simulink model "sig_mod_block_6"  (R2019a)
settings: Solver=VariableStepAuto  StartTime=0.0  StopTime=10.0  RelTol=1e-3
undefined symbols (not defined in the file): mod_fcn, sig_in, sig_mod_enabled, sig_out
libraries: simulink x3
settings Model: Creator=a3bawa  LastModifiedBy=a3bawa

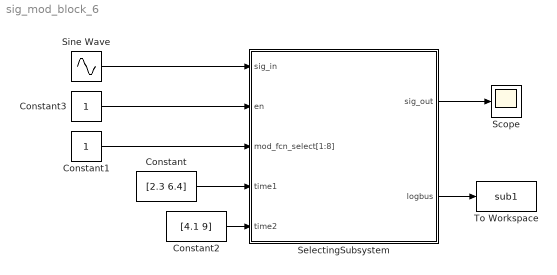
== system sig_mod_block_6 ==
  Constant : Constant  Value=[2.3 6.4]
  Constant1 : Constant
  Constant2 : Constant  Value=[4.1 9]
  Constant3 : Constant
  Scope : Scope
  SelectingSubsystem : Subsystem
  Sine Wave : Sin  SampleTime=0
  To Workspace : ToWorkspace  VariableName=sub1  SaveFormat=Timeseries  SampleTime=-1
  wires:
  Sine Wave/1 -> SelectingSubsystem/1(sig_in)
  Constant3/1 -> SelectingSubsystem/2(en)
  Constant1/1 -> SelectingSubsystem/3(mod_fcn_select[1:8])
  SelectingSubsystem/1(sig_out) -> Scope/1
  SelectingSubsystem/2(logbus) -> To Workspace/1
  Constant/1 -> SelectingSubsystem/4(time1)
  Constant2/1 -> SelectingSubsystem/5(time2)

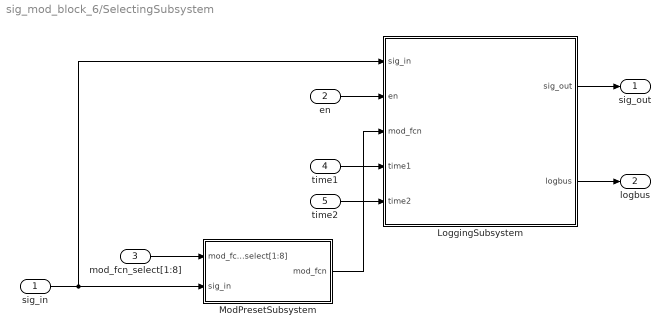
== system sig_mod_block_6/SelectingSubsystem ==
  sig_in : Inport
  en : Inport  Port=2
  mod_fcn_select[1:8] : Inport  Port=3
  time1 : Inport  Port=4
  time2 : Inport  Port=5
  LoggingSubsystem : Subsystem
  ModPresetSubsystem : Subsystem
  sig_out : Outport
  logbus : Outport  Port=2
  wires:
  sig_in/1 -> ModPresetSubsystem/2(sig_in), LoggingSubsystem/1(sig_in)
  en/1 -> LoggingSubsystem/2(en)
  LoggingSubsystem/1(sig_out) -> sig_out/1
  time1/1 -> LoggingSubsystem/4(time1)
  time2/1 -> LoggingSubsystem/5(time2)
  LoggingSubsystem/2(logbus) -> logbus/1
  mod_fcn_select[1:8]/1 -> ModPresetSubsystem/1(mod_fcn_select[1:8])
  ModPresetSubsystem/1(mod_fcn) -> LoggingSubsystem/3(mod_fcn)

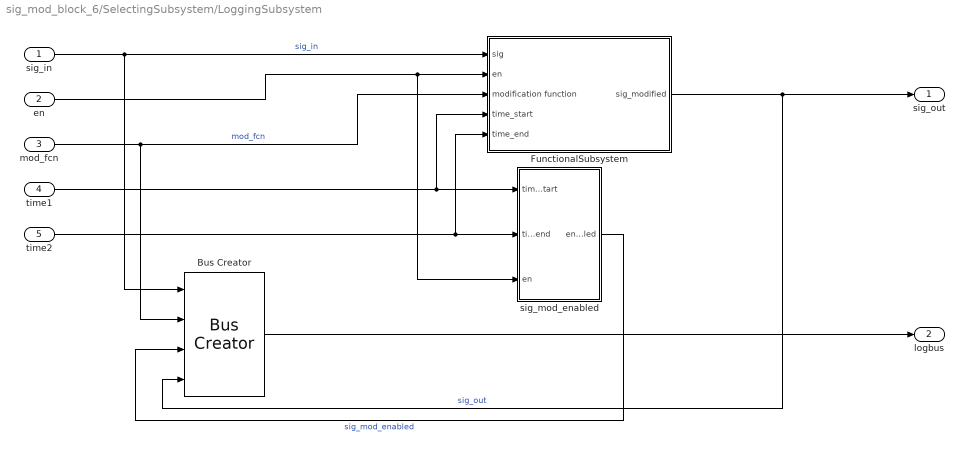
== system sig_mod_block_6/SelectingSubsystem/LoggingSubsystem ==
  sig_in : Inport
  en : Inport  Port=2
  mod_fcn : Inport  Port=3
  time1 : Inport  Port=4
  time2 : Inport  Port=5
  Bus Creator : BusCreator  Inputs=sig_in,mod_fcn,sig_mod_enabled,sig_out
  FunctionalSubsystem : Subsystem  TreatAsAtomicUnit=on
  sig_mod_enabled : Subsystem
  sig_out : Outport
  logbus : Outport  Port=2
  wires:
  FunctionalSubsystem/1(sig_modified) -> sig_out/1, Bus Creator/4  "sig_out"
  sig_in/1 -> FunctionalSubsystem/1(sig), Bus Creator/1  "sig_in"
  en/1 -> FunctionalSubsystem/2(en), sig_mod_enabled/3(en)
  sig_mod_enabled/1(enabled) -> Bus Creator/3  "sig_mod_enabled"
  mod_fcn/1 -> FunctionalSubsystem/3(modification function), Bus Creator/2  "mod_fcn"
  time1/1 -> sig_mod_enabled/1(time_start), FunctionalSubsystem/4(time_start)
  time2/1 -> FunctionalSubsystem/5(time_end), sig_mod_enabled/2(time_end)
  Bus Creator/1 -> logbus/1

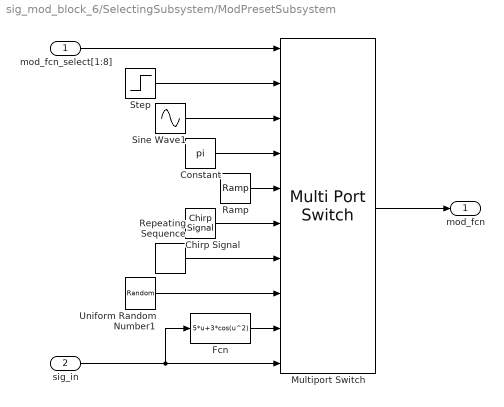
== system sig_mod_block_6/SelectingSubsystem/ModPresetSubsystem ==
  mod_fcn_select[1:8] : Inport
  sig_in : Inport  Port=2
  Chirp Signal : simulink/Sources/Chirp Signal  f1=1  T=10  f2=1000
  Constant : Constant  Value=pi
  Fcn : Fcn  Expr=5*u+3*cos(u^2)
  Multiport Switch : MultiPortSwitch  Inputs=8  DataPortForDefault=Additional data port  DiagnosticForDefault=Warning
  Ramp : simulink/Sources/Ramp  slope=1  start=5  InitialOutput=0
  Repeating Sequence : simulink/Sources/Repeating Sequence  rep_seq_t=[0 2]  rep_seq_y=[0 1]
  Sine Wave1 : Sin  Frequency=1000  SampleTime=0
  Step : Step  Time=5  SampleTime=0
  Uniform Random Number1 : UniformRandomNumber  SampleTime=0.1
  mod_fcn : Outport
  wires:
  mod_fcn_select[1:8]/1 -> Multiport Switch/1
  Step/1 -> Multiport Switch/2
  Chirp Signal/1 -> Multiport Switch/6
  sig_in/1 -> Fcn/1, Multiport Switch/10
  Fcn/1 -> Multiport Switch/9
  Sine Wave1/1 -> Multiport Switch/3
  Uniform Random Number1/1 -> Multiport Switch/8
  Ramp/1 -> Multiport Switch/5
  Repeating Sequence/1 -> Multiport Switch/7
  Constant/1 -> Multiport Switch/4
  Multiport Switch/1 -> mod_fcn/1

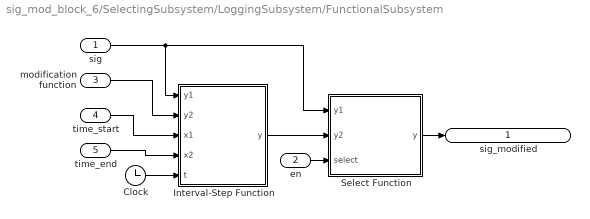
== system sig_mod_block_6/SelectingSubsystem/LoggingSubsystem/FunctionalSubsystem ==
  sig : Inport
  en : Inport  Port=2
  modification function : Inport  Port=3
  time_start : Inport  Port=4
  time_end : Inport  Port=5
  Clock : Clock
  Interval-Step Function : MATLAB Function  TreatAsAtomicUnit=on
  Select Function : MATLAB Function  TreatAsAtomicUnit=on
  sig_modified : Outport
  wires:
  Interval-Step Function/1(y) -> Select Function/2(y2)
  Clock/1 -> Interval-Step Function/5(t)
  en/1 -> Select Function/3(select)
  sig/1 -> Interval-Step Function/1(y1), Select Function/1(y1)
  Select Function/1(y) -> sig_modified/1
  modification function/1 -> Interval-Step Function/2(y2)
  time_start/1 -> Interval-Step Function/3(x1)
  time_end/1 -> Interval-Step Function/4(x2)

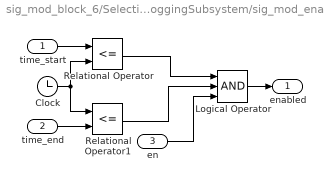
== system sig_mod_block_6/SelectingSubsystem/LoggingSubsystem/sig_mod_enabled ==
  time_start : Inport
  time_end : Inport  Port=2
  en : Inport  Port=3
  Clock : Clock
  Logical Operator : Logic  Inputs=3  AllPortsSameDT=off  OutDataTypeStr=boolean
  Relational Operator : RelationalOperator  Operator=<=  OutDataTypeStr=boolean  RndMeth=Simplest
  Relational Operator1 : RelationalOperator  Operator=<=  OutDataTypeStr=boolean  RndMeth=Simplest
  enabled : Outport
  wires:
  Relational Operator1/1 -> Logical Operator/2
  Clock/1 -> Relational Operator1/1, Relational Operator/2
  time_end/1 -> Relational Operator1/2
  Relational Operator/1 -> Logical Operator/1
  time_start/1 -> Relational Operator/1
  Logical Operator/1 -> enabled/1
  en/1 -> Logical Operator/3

== matlab function sig_mod_block_6/SelectingSubsystem/LoggingSubsystem/FunctionalSubsystem/Interval-Step Function ==
  data: y1 input; y output; y2 input; x1 input; x2 input; t input
function y = fcn(y1,y2,x1,x2,t)

if length(x1)~=length(x2)
    error('Interval-Step Function Error: time1 vector and time2 vector are not same length');
end
y=y1;
for i=1:1:length(x1)
    if (x1(i)<=t)&&(t<x2(i))
        y=y2;
    end
end

== matlab function sig_mod_block_6/SelectingSubsystem/LoggingSubsystem/FunctionalSubsystem/Select Function ==
  data: y1 input; y output; y2 input; select input
function y = fcn(y1,y2,select)

if select>=1
    y=y2;
else
    y=y1;
end
